simulink model "automata_learning"  (R2022a)
settings: Solver=FixedStepAuto  StartTime=0.0  StopTime=10.0  FixedStep=0.01  RelTol=1e-3
(part 2 of 10)

== stateflow chart automata_learning/automata_learning ==
  settings: updateMethod=CONTINUOUS
  state loc1
    du:
